simulink model "DEA_a"  (R2018a)
settings: Solver=ode15s  StartTime=0.0  StopTime=100  EnableMultiTasking=on
InitFcn:
  | Parameter;
settings Model: Creator=Johannes  LastModifiedBy=Matthias
settings DataIOCC: LimitDataPoints=on  SaveFormat=Array  SignalLoggingSaveFormat=ModelDataLogs
settings OptimizationCC: LifeSpan=inf
settings DebuggingCC: UnderspecifiedInitializationDetection=Classic  MergeDetectMultiDrivingBlocksExec=none  SolverPrmCheckMsg=warning  MultiTaskDSMMsg=warning  MultiTaskCondExecSysMsg=none  SFUnexpectedBacktrackingDiag=warning  SFNoUnconditionalDefaultTransitionDiag=warning  SFExecutionAtInitializationDiag=none
settings HardwareCC: ProdBitPerPointer=32  ProdBitPerSizeT=32  ProdBitPerPtrDiffT=32  ProdLargestAtomicFloat=None  ProdIntDivRoundTo=Undefined  ProdEndianess=Unspecified  ProdWordSize=32  ProdHWDeviceType=32-bit Generic
settings ModelReferenceCC: PropagateSignalLabelsOutOfModel=off
settings CodeAppCC: StateflowObjectComments=on
settings GRTTargetCC: TargetLangStandard=C89/C90 (ANSI)  GeneratePreprocessorConditionals=Disable all
settings ConfigComp: CovMetricSettings=dw  CovHtmlReporting=on  CovSaveCumulativeToWorkspaceVar=on  CovSaveSingleToWorkspaceVar=on  CovExternalEMLEnable=off

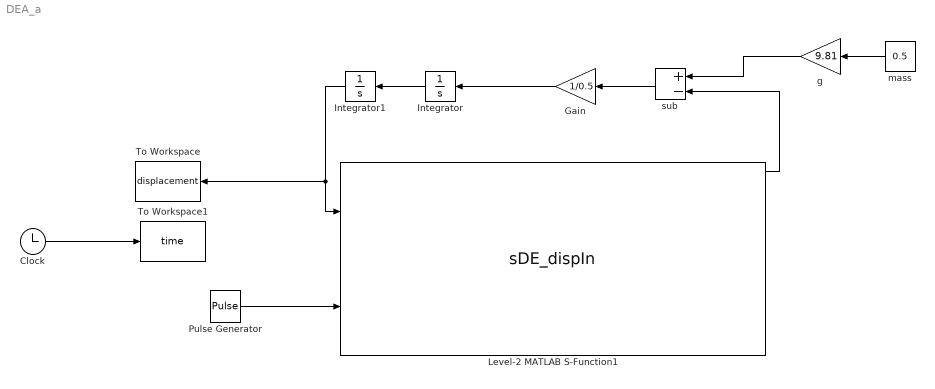
== system DEA_a ==
  Clock : Clock
  Gain : Gain  Gain=1/0.5
  Integrator : Integrator
  Integrator1 : Integrator  InitialCondition=0.066
  Level-2 MATLAB S-Function1 : M-S-Function  FunctionName=sDE_dispIn  Parameters=params, initConds
      mask Display:
      | color('black');
      | patch(4*[-1 1 1 -1],1.75*[-1 -1 1 1],[1 1 1]);
      | patch(2*[-1 1 1 -1],1.2*[-1 -1 1 1],[0 0 0]);
      | patch(1.95*[-1 1 1 -1],0.8*[-1 -1 1 1],[1 1 1]);
      | disp('DE Actuator');
      | 
      | color('blue');
      | port_label('input', 1, 'y [m]','texmode','on');
      | port_label('input', 2, 'v [V]','texmode','on');
      | 
      | color('red');
      | port_label('output', 1, 'F [N]','texmode','on');
      | port_label('output', 2, 'x_v [-]','texmode','on');
      | port_label('output', 3, 'q [C]','texmode','on');
      | port_label('output', 4, '\epsilon_1 [-]','texmode','on');
      | port_label('output', 5, '\sigma_1 [Pa]','texmode','on');
      | port_label('output', 6, 'i [A]','texmode','on');
      | port_label('output', 7, 'v_{DE} [V]','texmode','on');
      | port_label('output', 8, 'C [F]','texmode','on');
  Pulse Generator : DiscretePulseGenerator  PulseType=Time based  Amplitude=2500  Period=10  PulseWidth=50
  To Workspace : ToWorkspace  VariableName=displacement  SampleTime=-1
  To Workspace1 : ToWorkspace  VariableName=time  SampleTime=-1
  g : Gain  Gain=9.81
  mass : Constant  Value=0.5
  sub : Sum  Inputs=+-
  wires:
  mass/1 -> g/1
  g/1 -> sub/1
  Level-2 MATLAB S-Function1/1 -> sub/2
  sub/1 -> Gain/1
  Gain/1 -> Integrator/1
  Integrator/1 -> Integrator1/1
  Pulse Generator/1 -> Level-2 MATLAB S-Function1/2
  Integrator1/1 -> To Workspace/1, Level-2 MATLAB S-Function1/1
  Clock/1 -> To Workspace1/1
